simulink model "zadacha_13"  (Simulink 7.1)
settings: Solver=ode45  StartTime=0.0  StopTime=20  RelTol=1e-3
settings Model: Creator=Slavi  LastModifiedBy=Slavi

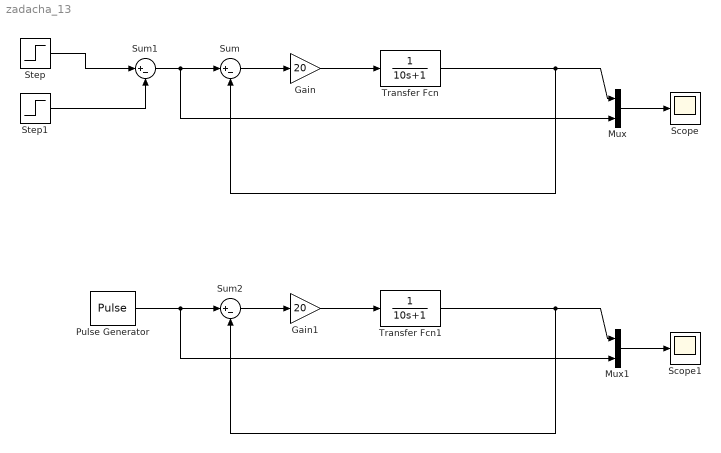
== system zadacha_13 ==
  Gain : Gain  Gain=20  ParameterDataType=sfix(16)  ParameterScaling=2^0  OutDataType=sfix(16)  OutScaling=2^0
  Gain1 : Gain  Gain=20  ParameterDataType=sfix(16)  ParameterScaling=2^0  OutDataType=sfix(16)  OutScaling=2^0
  Mux : Mux  Inputs=2
  Mux1 : Mux  Inputs=2
  Pulse Generator : DiscretePulseGenerator  PulseType=Time based  Period=1  PulseWidth=90
  Scope : Scope
  Scope1 : Scope
  Step : Step  Time=0
  Step1 : Step
  Sum : Sum  Inputs=|+-  OutDataType=sfix(16)  OutScaling=2^0
  Sum1 : Sum  Inputs=|+-  OutDataType=sfix(16)  OutScaling=2^0
  Sum2 : Sum  Inputs=|+-  OutDataType=sfix(16)  OutScaling=2^0
  Transfer Fcn : TransferFcn  Denominator=[10 1]
  Transfer Fcn1 : TransferFcn  Denominator=[10 1]
  wires:
  Transfer Fcn/1 -> Mux/1, Sum/2
  Gain/1 -> Transfer Fcn/1
  Sum1/1 -> Sum/1, Mux/2
  Sum/1 -> Gain/1
  Mux/1 -> Scope/1
  Step/1 -> Sum1/1
  Step1/1 -> Sum1/2
  Transfer Fcn1/1 -> Mux1/1, Sum2/2
  Gain1/1 -> Transfer Fcn1/1
  Pulse Generator/1 -> Sum2/1, Mux1/2
  Sum2/1 -> Gain1/1
  Mux1/1 -> Scope1/1
